simulink model "Problem_1"  (R2023b)
settings: Solver=VariableStepAuto  StartTime=0.0  StopTime=t  FixedStep=dt  RelTol=1e-3
values from neighbouring files (symbols this model uses):
  A1 = 1    [Problem_1_script.m]
  A2 = .1    (= 0.1)    [Problem_1_script.m]
  alpha = 1    [Problem_1_script.m]
  beta = 0.003    [Problem_1_script.m]
  g = 9.81    [Problem_1_script.m]
  Gamma = [ g11 g12 g13 ... (first row only)    [Problem_1_script.m]
  l = 1    [Problem_1_script.m]
  lambda_0 = (lambda_1/2)^2    (= 4)    [Problem_1_script.m]
  lambda_1 = 2*k    (= 4)    [Problem_1_script.m]
  m = 0.2    [Problem_1_script.m]
  theta_0 = [1/(m_0*l_0^2) beta_0/(m_0*l_0^2) 1/l_0]'    [Problem_1_script.m]
  w1 = pi    (= 3.14159265359)    [Problem_1_script.m]
  w2 = pi*.3    (= 0.942477796077)    [Problem_1_script.m]
undefined symbols (not defined in the file or in its folder): K
settings Model: Creator=eliasoa  LastModifiedBy=Elias
settings OptimizationCC: BlockReduction=off  DefaultParameterBehavior=Inlined  BufferReuse=off

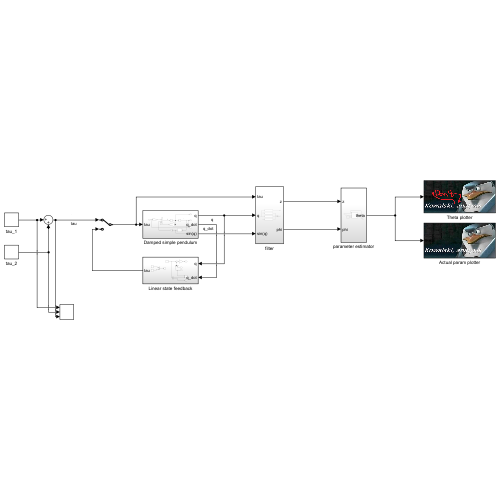
[thumbnail: Simulink's stored preview of the top-level diagram]
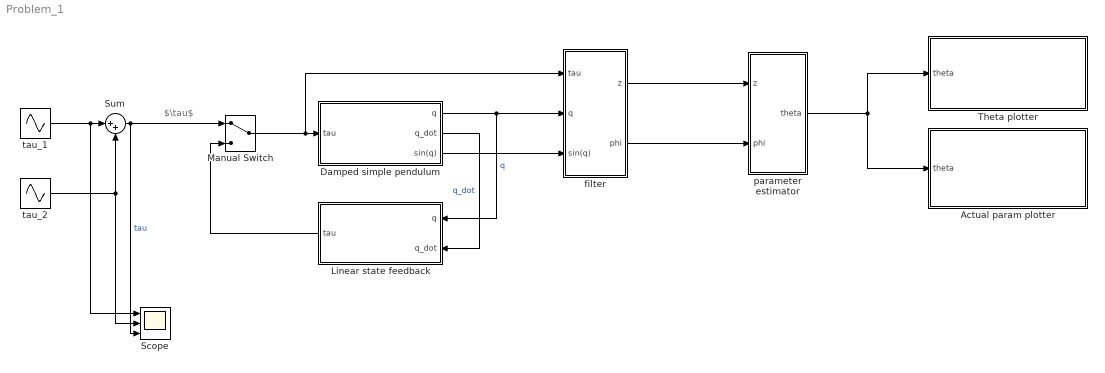
== system Problem_1 ==
  note: $\tau$
  Actual param plotter : Subsystem
      mask Display: image('Kowalski.jpg'); % Use "Edit Image" on toolstrip to change.
  Damped simple pendulum : Subsystem
  Linear state feedback : Subsystem
  Manual Switch : ManualSwitch
  Scope : Scope  NumInputPorts=3
  Sum : Sum  Inputs=|++
  Theta plotter : Subsystem
      mask Display: image('Kowalski dont.jpg'); % Use "Edit Image" on toolstrip to change.
  filter : Subsystem
  parameter estimator : Subsystem
  tau_1 : Sin  Amplitude=A1  Frequency=w1  SampleTime=0
  tau_2 : Sin  Amplitude=A2  Frequency=w2  SampleTime=0
  wires:
  Damped simple pendulum/3(sin(q)) -> filter/3(sin(q))
  Damped simple pendulum/1(q) -> Linear state feedback/1(q), filter/2(q)  "q"
  filter/2(phi) -> parameter estimator/2(phi)
  filter/1(z) -> parameter estimator/1(z)
  parameter estimator/1(theta) -> Theta plotter/1(theta), Actual param plotter/1(theta)
  Manual Switch/1 -> filter/1(tau), Damped simple pendulum/1(tau)
  Damped simple pendulum/2(q_dot) -> Linear state feedback/2(q_dot)  "q_dot"
  Linear state feedback/1(tau) -> Manual Switch/2
  Sum/1 -> Scope/3, Manual Switch/1  "tau"
  tau_2/1 -> Scope/2, Sum/2
  tau_1/1 -> Scope/1, Sum/1

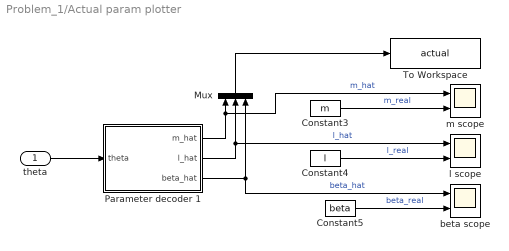
== system Problem_1/Actual param plotter ==
  theta : Inport
  Constant3 : Constant  Value=m
  Constant4 : Constant  Value=l
  Constant5 : Constant  Value=beta
  Mux : Mux  Inputs=3
  Parameter decoder 1 : MATLAB Function  TreatAsAtomicUnit=on
  To Workspace : ToWorkspace  VariableName=actual  SaveFormat=Timeseries  SampleTime=-1
  beta scope : Scope  NumInputPorts=2
  l scope : Scope  NumInputPorts=2
  m scope : Scope  NumInputPorts=2
  wires:
  Parameter decoder 1/2(l_hat) -> l scope/1, Mux/2  "l_hat"
  Constant5/1 -> beta scope/2  "beta_real"
  theta/1 -> Parameter decoder 1/1(theta)
  Constant3/1 -> m scope/2  "m_real"
  Parameter decoder 1/1(m_hat) -> m scope/1, Mux/1  "m_hat"
  Parameter decoder 1/3(beta_hat) -> beta scope/1, Mux/3  "beta_hat"
  Constant4/1 -> l scope/2  "l_real"
  Mux/1 -> To Workspace/1

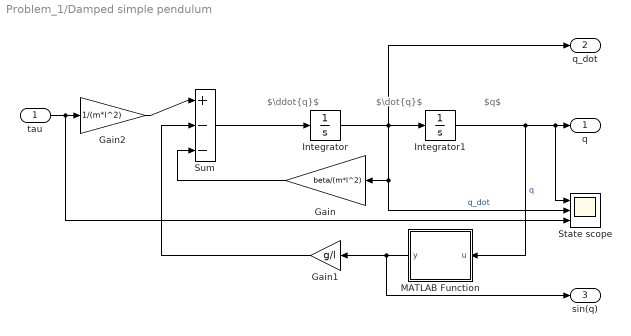
== system Problem_1/Damped simple pendulum ==
  note: $\ddot{q}$
  note: $\dot{q}$
  note: $q$
  tau : Inport
  Gain : Gain  Gain=beta/(m*l^2)
  Gain1 : Gain  Gain=g/l
  Gain2 : Gain  Gain=1/(m*l^2)
  Integrator : Integrator
  Integrator1 : Integrator
  MATLAB Function : MATLAB Function  TreatAsAtomicUnit=on
  State scope : Scope  NumInputPorts=3
  Sum : Sum  Inputs=|+--
  q : Outport
  q_dot : Outport  Port=2
  sin(q) : Outport  Port=3
  wires:
  tau/1 -> State scope/3, Gain2/1
  Sum/1 -> Integrator/1
  Gain2/1 -> Sum/1
  Gain/1 -> Sum/3
  MATLAB Function/1(y) -> Gain1/1, sin(q)/1
  Gain1/1 -> Sum/2
  Integrator/1 -> Integrator1/1, q_dot/1, State scope/2, Gain/1  "q_dot"
  Integrator1/1 -> MATLAB Function/1(u), State scope/1, q/1  "q"

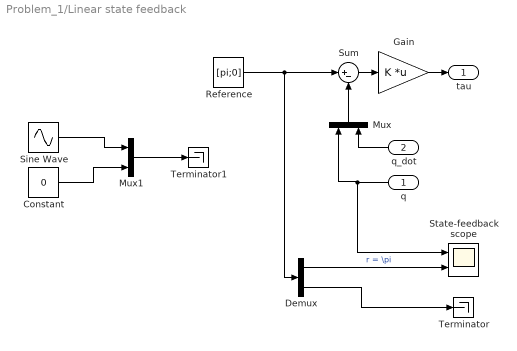
== system Problem_1/Linear state feedback ==
  q : Inport
  q_dot : Inport  Port=2
  Constant : Constant  Value=0
  Demux : Demux  Outputs=2
  Gain : Gain  Gain=K  Multiplication=Matrix(K*u)
  Mux : Mux  Inputs=2
  Mux1 : Mux  Inputs=2
  Reference : Constant  Value=[pi;0]
  Sine Wave : Sin  Frequency=.1  SampleTime=0
  State-feedback scope : Scope  NumInputPorts=2
  Sum : Sum  Inputs=|+-
  Terminator : Terminator
  Terminator1 : Terminator
  tau : Outport
  wires:
  Sum/1 -> Gain/1
  Mux/1 -> Sum/2
  Demux/2 -> Terminator/1
  q_dot/1 -> Mux/2
  q/1 -> Mux/1, State-feedback scope/1
  Demux/1 -> State-feedback scope/2  "r = \\pi"
  Gain/1 -> tau/1
  Constant/1 -> Mux1/2
  Sine Wave/1 -> Mux1/1
  Reference/1 -> Demux/1, Sum/1
  Mux1/1 -> Terminator1/1

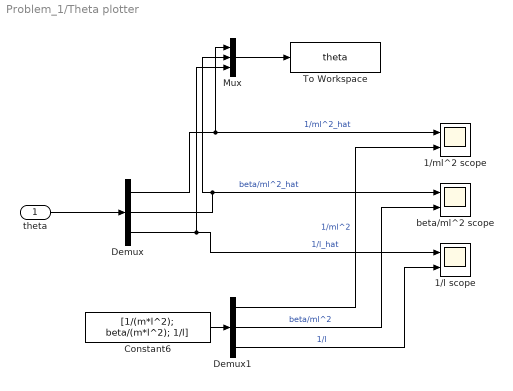
== system Problem_1/Theta plotter ==
  theta : Inport
  1/l scope : Scope  NumInputPorts=2
  1/ml^2 scope : Scope  NumInputPorts=2
  Constant6 : Constant  Value=[1/(m*l^2); beta/(m*l^2); 1/l]
  Demux : Demux  Outputs=3
  Demux1 : Demux  Outputs=3
  Mux : Mux  Inputs=3
  To Workspace : ToWorkspace  VariableName=theta  SaveFormat=Timeseries  SampleTime=-1
  beta/ml^2 scope : Scope  NumInputPorts=2
  wires:
  Demux/2 -> Mux/2, beta/ml^2 scope/1  "beta/ml^2_hat"
  Demux1/1 -> 1/ml^2 scope/2  "1/ml^2"
  Demux/1 -> Mux/1, 1/ml^2 scope/1  "1/ml^2_hat"
  Constant6/1 -> Demux1/1
  Demux1/3 -> 1/l scope/2  "1/l"
  theta/1 -> Demux/1
  Demux1/2 -> beta/ml^2 scope/2  "beta/ml^2"
  Demux/3 -> 1/l scope/1, Mux/3  "1/l_hat"
  Mux/1 -> To Workspace/1

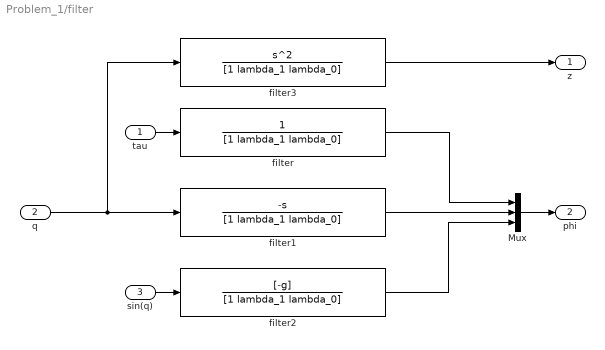
== system Problem_1/filter ==
  tau : Inport
  q : Inport  Port=2
  sin(q) : Inport  Port=3
  Mux : Mux  Inputs=3
  filter : TransferFcn  Denominator=[1 lambda_1 lambda_0]
  filter1 : TransferFcn  Numerator=[-1 0]  Denominator=[1 lambda_1 lambda_0]
  filter2 : TransferFcn  Numerator=[-g]  Denominator=[1 lambda_1 lambda_0]
  filter3 : TransferFcn  Numerator=[1 0 0]  Denominator=[1 lambda_1 lambda_0]
  z : Outport
  phi : Outport  Port=2
  wires:
  filter1/1 -> Mux/2
  filter2/1 -> Mux/3
  filter/1 -> Mux/1
  sin(q)/1 -> filter2/1
  tau/1 -> filter/1
  q/1 -> filter3/1, filter1/1
  Mux/1 -> phi/1
  filter3/1 -> z/1

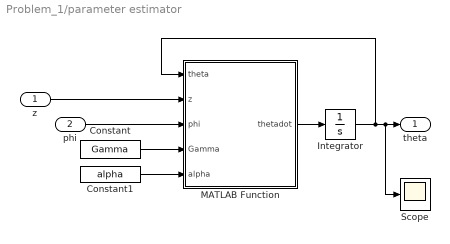
== system Problem_1/parameter estimator ==
  z : Inport
  phi : Inport  Port=2
  Constant : Constant  Value=Gamma
  Constant1 : Constant  Value=alpha
  Integrator : Integrator  InitialCondition=theta_0
  MATLAB Function : MATLAB Function  TreatAsAtomicUnit=on
  Scope : Scope
  theta : Outport
  wires:
  Constant1/1 -> MATLAB Function/5(alpha)
  Integrator/1 -> Scope/1, theta/1, MATLAB Function/1(theta)
  phi/1 -> MATLAB Function/3(phi)
  MATLAB Function/1(thetadot) -> Integrator/1
  z/1 -> MATLAB Function/2(z)
  Constant/1 -> MATLAB Function/4(Gamma)

== matlab function Problem_1/Damped simple pendulum/MATLAB Function ==
  data: u input; y output
function y = sin(u)

y = sin(u);

== matlab function Problem_1/parameter estimator/MATLAB Function ==
  data: theta input; thetadot output; z input; phi input; Gamma input; alpha input
function thetadot = fcn(theta,z,phi,Gamma,alpha)
m2 = 1 + alpha*(phi'*phi);
epsilon = (z-theta'*phi)/m2;
thetadot = Gamma * epsilon * phi;

== matlab function Problem_1/Actual param plotter/Parameter decoder 1 ==
  data: theta input; m_hat output; l_hat output; beta_hat output
function [m_hat,l_hat,beta_hat] = fcn(theta)
theta_1 = theta(1); %  1 / ml^2
theta_2 = theta(2); % β / ml^2
theta_3 = theta(3); % 1 / l

m_hat= theta_3^2/(theta_1);
l_hat = 1/theta_3;
beta_hat= theta_2/theta_1;
